simulink model "dev_RigTest_networkOnly"  (R2020b)
settings: Solver=VariableStepAuto  StartTime=0.0  StopTime=1500  RelTol=1e-3
libraries: IMT_Library x3, simulink_extras x2, slpidlib x1
settings Model: Creator=Mr_Li  LastModifiedBy=Mr_Li

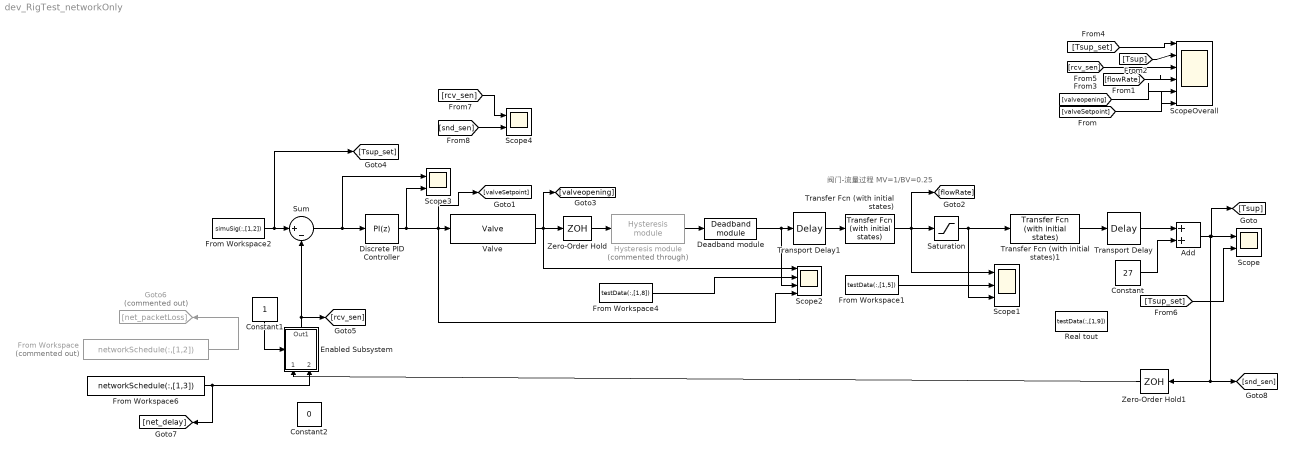
== system dev_RigTest_networkOnly ==
  note: 阀门-流量过程
      | MV=1/BV=0.25
  Add : Sum
  Constant : Constant  Value=27
  Constant1 : Constant
  Constant2 : Constant  Value=0
  Deadband module : IMT_Library/Deadband module  upper=22.5  lower=6.5
      settings: SourceProductName=Imitation
  Discrete PID Controller : slpidlib/PID Controller  Controller=PI  Form=Parallel  TimeDomain=Discrete-time  UseExternalTs=off  SampleTime=1  IntegratorMethod=Forward Euler  FilterMethod=Forward Euler  ControllerParametersSource=internal  P=0.5  I=0.00715  D=0  UseFilter=on  N=100  TunerSelectOption=Frequency Response Based  InitialConditionSource=internal  InitialConditionForIntegrator=0  InitialConditionForFilter=0  DifferentiatorICPrevScaledInput=0  ExternalReset=none  TrackingMode=off  Kt=1  LimitOutput=off  SatLimitsSource=internal  UpperSaturationLimit=inf  LowerSaturationLimit=-inf  LinearizeAsGain=off  AntiWindupMode=none  Kb=1  POutMin=[]  POutMax=[]  IOutMin=[]  IOutMax=[]  DOutMin=[]  DOutMax=[]  NOutMin=[]  NOutMax=[]  SumOutMin=[]  SumOutMax=[]  SaturationOutMin=[]  SaturationOutMax=[]  PParamMin=[]  PParamMax=[]  IParamMin=[]  IParamMax=[]  DParamMin=[]  DParamMax=[]  NParamMin=[]  NParamMax=[]  KbParamMin=[]  KbParamMax=[]  KtParamMin=[]  KtParamMax=[]  KbOutMin=[]  KbOutMax=[]  KtOutMin=[]  KtOutMax=[]  IntegratorOutMin=[]  IntegratorOutMax=[]  FilterOutMin=[]  FilterOutMax=[]  SumI1OutMin=[]  SumI1OutMax=[]  SumI2OutMin=[]  SumI2OutMax=[]  SumI3OutMin=[]  SumI3OutMax=[]  SumI4OutMin=[]  SumI4OutMax=[]  SumDOutMin=[]  SumDOutMax=[]  DifferentiatorOutMin=[]  DifferentiatorOutMax=[]  FilterDiffOutCoefMin=[]  FilterDiffOutCoefMax=[]  ReciprocalOutMin=[]  ReciprocalOutMax=[]  SumDenOutMin=[]  SumDenOutMax=[]  SumNumOutMin=[]  SumNumOutMax=[]  DivideOutMin=[]  DivideOutMax=[]  UdiffTsProdOutMin=[]  UdiffTsProdOutMax=[]  NTsProdOutMin=[]  NTsProdOutMax=[]  UintegralTsProdOutMin=[]  UintegralTsProdOutMax=[]  UngainTsProdOutMin=[]  UngainTsProdOutMax=[]  IntegratorContinuousStateAttributes=''  IntegratorStateMustResolveToSignalObject=off  IntegratorRTWStateStorageClass=Auto  FilterContinuousStateAttributes=''  FilterStateMustResolveToSignalObject=off  FilterRTWStateStorageClass=Auto  ParallelPVariant=InternalParameters  IdealPVariant=Disabled  IVariant=InternalParameters  DVariant=Disabled  IntegratorVariant=Discrete  SatVariant=Disabled  AWVariant=Passthrough  PCopyVariant=Disabled  TRVariant=Disabled  FdbkBlocksVariant=Forward  IdealPFdbkVariant=Disabled  SatFdbkVariant=Disabled  DerivativeFilterVariant=Disabled  NVariant=Disabled  NCopyVariant=Disabled_SignalSpec  FilterICVariant=Disabled  IntegratorICVariant=InternalICs  ExternalResetVariant=Disabled  TRSumVariant=Passthrough  SumFdbkVariant=Disabled  SumVariant=Sum_PI  TsampFilterVariant=InternalTs  TsampNgainVariant=Passthrough  TsampIntegralVariant=Passthrough  ExternalSaturationOutDataTypeStr=Inherit: Same as second input
  Enabled Subsystem : Subsystem  TreatAsAtomicUnit=on
  From Workspace : FromWorkspace  Commented=on  VariableName=networkSchedule(:,[1,2])  SampleTime=1
  From Workspace1 : FromWorkspace  VariableName=testData(:,[1,5])
  From Workspace2 : FromWorkspace  VariableName=simuSig(:,[1,2])  SampleTime=1
  From Workspace4 : FromWorkspace  VariableName=testData(:,[1,8])  SampleTime=1
  From Workspace6 : FromWorkspace  VariableName=networkSchedule(:,[1,3])  OutDataTypeStr=double  SampleTime=0.001  OutputAfterFinalValue=Holding final value
  Goto6 : Goto  Commented=on  GotoTag=net_packetLoss
  Hysteresis module : IMT_Library/Hysteresis module  Commented=through  hysteresisSize=4.5
      settings: SourceProductName=Imitation
  Real tout : FromWorkspace  VariableName=testData(:,[1,9])
  Saturation : Saturate  UpperLimit=0.25  LowerLimit=0
  Scope : Scope  NumInputPorts=2
  Scope1 : Scope  NumInputPorts=3
  Scope2 : Scope  NumInputPorts=4
  Scope3 : Scope  NumInputPorts=2
  Scope4 : Scope  NumInputPorts=2
  ScopeOverall : Scope  NumInputPorts=6
  Sum : Sum  Inputs=|+-
  Transfer Fcn (with initial states) : simulink_extras/Additional Linear/Transfer Fcn (with initial states)  N=[0.032]  D=[3.6 1]  X0=0
  Transfer Fcn (with initial states)1 : simulink_extras/Additional Linear/Transfer Fcn (with initial states)  N=[105]  D=[380 40 1]  X0=0
  Transport Delay : TransportDelay  DelayTime=0
  Transport Delay1 : TransportDelay  DelayTime=3
  Valve : IMT_Library/Valve  upper=101  lower=1.2  movementThreshold=1
      settings: SourceProductName=Imitation
  Zero-Order Hold : ZeroOrderHold
  Zero-Order Hold1 : ZeroOrderHold
  wires:
  Hysteresis module/1 -> Deadband module/1
  Constant/1 -> Add/2
  Transport Delay1/1 -> Transfer Fcn (with initial states)/1
  Valve/1 -> [valveopening], Scope2/1, Zero-Order Hold/1
  Transfer Fcn (with initial states)/1 -> Saturation/1, [flowRate], Scope1/1
  Discrete PID Controller/1 -> Valve/1, Scope2/4, [valveSetpoint], Scope3/2
  Sum/1 -> Scope3/1, Discrete PID Controller/1
  From Workspace1/1 -> Scope1/2
  Saturation/1 -> Scope1/3, Transfer Fcn (with initial states)1/1
  Deadband module/1 -> Scope2/3, Transport Delay1/1
  From Workspace4/1 -> Scope2/2
  Zero-Order Hold/1 -> Hysteresis module/1
  Transport Delay/1 -> Add/1
  Transfer Fcn (with initial states)1/1 -> Transport Delay/1
  From Workspace6/1 -> Enabled Subsystem/2(delay), [net_delay]
  Add/1 -> Zero-Order Hold1/1, [snd_sen], Scope/1, [Tsup]
  From Workspace/1 -> Goto6/1
  [Tsup_set] -> Scope/2
  From Workspace2/1 -> [Tsup_set], Sum/1
  [Tsup_set] -> ScopeOverall/1
  [Tsup] -> ScopeOverall/2
  [rcv_sen] -> ScopeOverall/3
  [flowRate] -> ScopeOverall/4
  [valveopening] -> ScopeOverall/5
  [valveSetpoint] -> ScopeOverall/6
  Zero-Order Hold1/1 -> Enabled Subsystem/1(data)
  [snd_sen] -> Scope4/2
  [rcv_sen] -> Scope4/1
  Enabled Subsystem/1(Out1) -> Sum/2, [rcv_sen]
  Constant1/1 -> Enabled Subsystem/Enable

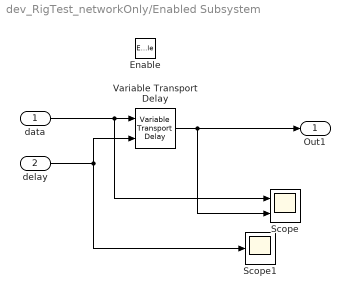
== system dev_RigTest_networkOnly/Enabled Subsystem ==
  data : Inport
  delay : Inport  Port=2
  Enable : EnablePort
  Scope : Scope  NumInputPorts=2
  Scope1 : Scope
  Variable Transport Delay : VariableTransportDelay  MaximumDelay=10  MaximumPoints=4000  ZeroDelay=on
  Out1 : Outport
  wires:
  data/1 -> Variable Transport Delay/1, Scope/1
  delay/1 -> Variable Transport Delay/2, Scope1/1
  Variable Transport Delay/1 -> Out1/1, Scope/2
